simulink model "lump_model_v5_23b"  (R2023b)
settings: Solver=VariableStepAuto  StartTime=0.0  StopTime=1000  RelTol=1e-3
model workspace (MAT data in the model file):
  A_busbar = 0.0015
  A_pack = 0.711626248
  C_nominal = 3
  I_max = 157.708978328
  P = 5
  S = 138
  SoC_initial = 1
  T_amb = 318.15
  W_max = 38.1424148607
  busbar_CC_area = 0.000108
  busbar_Cp = 237
  busbar_length = 0.032
  busbar_mass = 0.01
  busbar_resistivity = 1.68e-08
  busbar_thermalcontact_resistance = 1
  cell_Cp = 1000
  cell_mass = 0.046
  h_busbar = 5
  h_pack = 7.83952040581
(part 3 of 3)

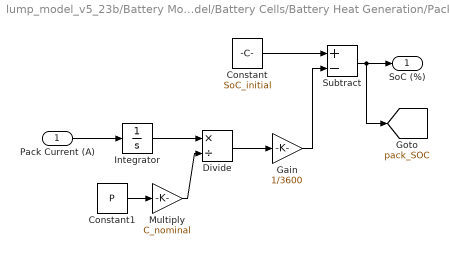
== system lump_model_v5_23b/Battery Model/Battery Cells/Battery Heat Generation/Pack SoC ==
  Pack Current (A) : Inport
  Constant : Constant  Value=SoC_initial
  Constant1 : Constant  Value=P
  Divide : Product  Inputs=*/
  Gain : Gain  Gain=1/3600
  Integrator : Integrator
  Multiply : Gain  Gain=C_nominal
  Subtract : Sum  Inputs=+-
  SoC (%) : Outport
  tag scope: pack_SOC=global
  wires:
  Pack Current (A)/1 -> Integrator/1
  Constant/1 -> Subtract/1
  Integrator/1 -> Divide/1
  Subtract/1 -> [pack_SOC], SoC (%)/1
  Constant1/1 -> Multiply/1
  Multiply/1 -> Divide/2
  Divide/1 -> Gain/1
  Gain/1 -> Subtract/2
